simulink model "IEEE_10_CIG_39bus"  (R2023b)
settings: Solver=ode23tb  StartTime=0.0  StopTime=10  MaxStep=1/60  RelTol=1e-2  AbsTol=1e-1  EnableMultiTasking=on
PreLoadFcn:
  | NE39bus_data;
  | PSSMODEL=1;
  | LPSS=0;
  | WAPSS=0;
  | WAPSS2=0;
undefined symbols (not defined in the file): D1, deg, Delta, kp, line, P_base, Pmax, Pmin, s, Udc, V_m
libraries: spsThreePhaseVIMeasurementLib x40, spsThreePhasePISectionLineLib x34, spsThreePhaseParallelRLCLoadLib x19, spsThreePhaseTransformerTwoWindingsLib x13, spsLoadFlowBusLib x10, spsMeanLib x10, spsPowerPositiveSequenceLib x10, spsDCVoltageSourceLib x10, spsUniversalBridgeLib x10, spsThreePhaseSeriesRLCBranchLib x2, spspowerguiLib x1
(part 2 of 2)

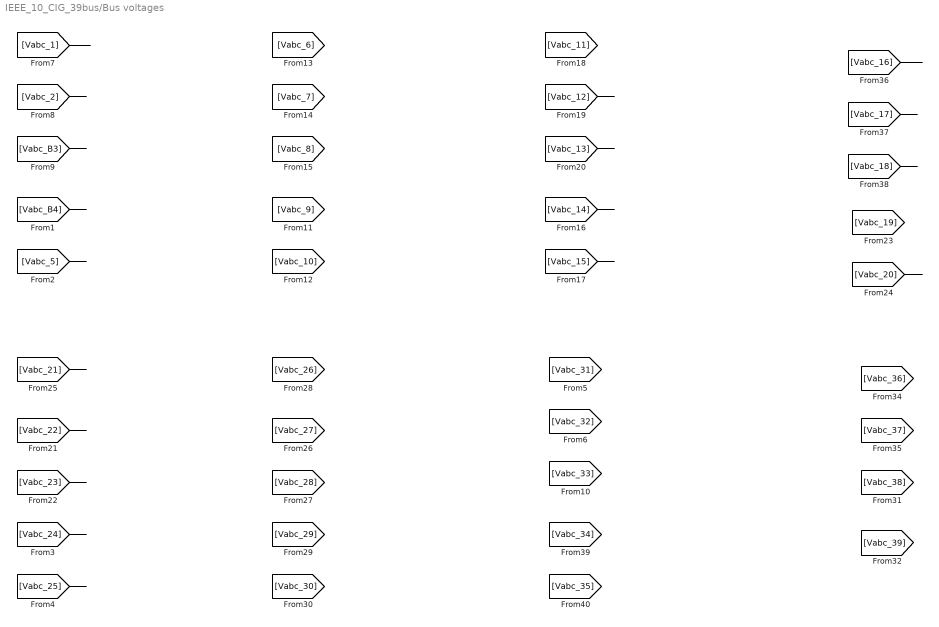
== system IEEE_10_CIG_39bus/Bus voltages ==
  wires:
  [Vabc_1] -> ?
  [Vabc_2] -> ?
  [Vabc_B3] -> ?
  [Vabc_B4] -> ?
  [Vabc_5] -> ?
  [Vabc_24] -> ?
  [Vabc_25] -> ?
  [Vabc_12] -> ?
  [Vabc_13] -> ?
  [Vabc_14] -> ?
  [Vabc_15] -> ?
  [Vabc_20] -> ?
  [Vabc_21] -> ?
  [Vabc_22] -> ?
  [Vabc_23] -> ?
  [Vabc_16] -> ?
  [Vabc_17] -> ?
  [Vabc_18] -> ?

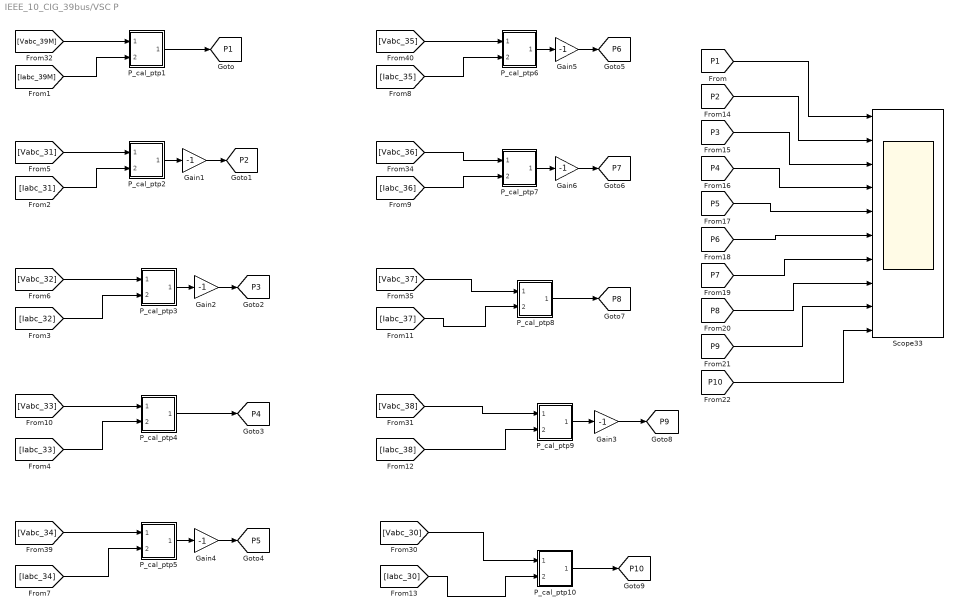
== system IEEE_10_CIG_39bus/VSC P ==
  Gain{1..6} (6 alike) : Gain  Gain=-1
  P_cal_ptp1 : Subsystem
  P_cal_ptp10 : Subsystem
  P_cal_ptp2 : Subsystem
  P_cal_ptp3 : Subsystem
  P_cal_ptp4 : Subsystem
  P_cal_ptp5 : Subsystem
  P_cal_ptp6 : Subsystem
  P_cal_ptp7 : Subsystem
  P_cal_ptp8 : Subsystem
  P_cal_ptp9 : Subsystem
  Scope33 : Scope  NumInputPorts=10
  tag scope: P10=global, P1=global, P2=global, P3=global, P4=global, P5=global, P6=global, P7=global, P8=global, P9=global
  wires:
  [Vabc_39M] -> P_cal_ptp1/1(In2)
  [Iabc_39M] -> P_cal_ptp1/2(In1)
  [Vabc_31] -> P_cal_ptp2/1(In2)
  [Iabc_31] -> P_cal_ptp2/2(In1)
  P_cal_ptp1/1(Out1) -> [P1]
  P_cal_ptp2/1(Out1) -> Gain1/1
  Gain1/1 -> [P2]
  [Vabc_32] -> P_cal_ptp3/1(In2)
  P_cal_ptp3/1(Out1) -> Gain2/1
  [Iabc_32] -> P_cal_ptp3/2(In1)
  Gain2/1 -> [P3]
  [Vabc_33] -> P_cal_ptp4/1(In2)
  [Iabc_33] -> P_cal_ptp4/2(In1)
  P_cal_ptp4/1(Out1) -> [P4]
  [Vabc_34] -> P_cal_ptp5/1(In2)
  P_cal_ptp5/1(Out1) -> Gain4/1
  [Iabc_34] -> P_cal_ptp5/2(In1)
  Gain4/1 -> [P5]
  [Vabc_35] -> P_cal_ptp6/1(In2)
  P_cal_ptp6/1(Out1) -> Gain5/1
  [Iabc_35] -> P_cal_ptp6/2(In1)
  Gain5/1 -> [P6]
  [Vabc_36] -> P_cal_ptp7/1(In2)
  P_cal_ptp7/1(Out1) -> Gain6/1
  [Iabc_36] -> P_cal_ptp7/2(In1)
  Gain6/1 -> [P7]
  [Iabc_37] -> P_cal_ptp8/2(In1)
  [Vabc_37] -> P_cal_ptp8/1(In2)
  P_cal_ptp8/1(Out1) -> [P8]
  [Vabc_38] -> P_cal_ptp9/1(In2)
  [Iabc_38] -> P_cal_ptp9/2(In1)
  P_cal_ptp10/1(Out1) -> [P10]
  [Vabc_30] -> P_cal_ptp10/1(In2)
  [Iabc_30] -> P_cal_ptp10/2(In1)
  [P1] -> Scope33/1
  [P2] -> Scope33/2
  [P3] -> Scope33/3
  [P4] -> Scope33/4
  [P5] -> Scope33/5
  [P6] -> Scope33/6
  [P7] -> Scope33/7
  [P8] -> Scope33/8
  [P9] -> Scope33/9
  [P10] -> Scope33/10
  P_cal_ptp9/1(Out1) -> Gain3/1
  Gain3/1 -> [P9]

== system IEEE_10_CIG_39bus/VSC1 ==
  DC Voltage Source2 : spsDCVoltageSourceLib/DC Voltage Source  Amplitude=Udc(1)  Measurements=None
  Memory2 : Memory
  Subsystem3 : Subsystem
  VSC1 : spsUniversalBridgeLib/Universal Bridge  Arms=3  SnubberResistance=1e5  SnubberCapacitance=inf  Device=Average-model based VSC  Ron=1e-3  Lon=0  ForwardVoltages="[  0  0  ]"  ForwardVoltage=0  GTOparameters=[ 10e-6 , 20e-6 ]  IGBTparameters=[ 1e-6 , 2e-6 ]  Measurements=None  Measurements_2=None  converterType=Rectifier
  Vref1 : Constant  Value=0
  A : PMIOPort  Side=Left
  B : PMIOPort  Port=2  Side=Left
  C : PMIOPort  Port=3  Side=Left
  wires:
  Subsystem3/2(Out2) -> [delta_P1]
  Memory2/1 -> VSC1/1
  [P1] -> Subsystem3/1(P2)
  Vref1/1 -> Subsystem3/2(delta)
  Subsystem3/1(Out1) -> Memory2/1
  connections:
  VSC1/LConn2 -- B/RConn1
  VSC1/RConn1 -- DC Voltage Source2/RConn1
  VSC1/RConn2 -- DC Voltage Source2/LConn1
  VSC1/LConn1 -- A/RConn1
  VSC1/LConn3 -- C/RConn1

== system IEEE_10_CIG_39bus/VSC2 ==
  DC Voltage Source1 : spsDCVoltageSourceLib/DC Voltage Source  Amplitude=Udc(2)  Measurements=None
  Memory1 : Memory
  Subsystem1 : Subsystem
  VSC2 : spsUniversalBridgeLib/Universal Bridge  Arms=3  SnubberResistance=1e5  SnubberCapacitance=inf  Device=Average-model based VSC  Ron=1e-3  Lon=0  ForwardVoltages="[  0  0  ]"  ForwardVoltage=0  GTOparameters=[ 10e-6 , 20e-6 ]  IGBTparameters=[ 1e-6 , 2e-6 ]  Measurements=None  Measurements_2=None  converterType=Rectifier
  Vref2 : Constant  Value=0
  A : PMIOPort  Side=Left
  B : PMIOPort  Port=2  Side=Left
  C : PMIOPort  Port=3  Side=Left
  wires:
  Subsystem1/2(Out2) -> [delta_P2]
  Subsystem1/1(Out1) -> Memory1/1
  Vref2/1 -> Subsystem1/2(delta)
  [P2] -> Subsystem1/1(P2)
  Memory1/1 -> VSC2/1
  connections:
  VSC2/LConn2 -- B/RConn1
  VSC2/RConn2 -- DC Voltage Source1/LConn1
  VSC2/RConn1 -- DC Voltage Source1/RConn1
  VSC2/LConn3 -- C/RConn1
  VSC2/LConn1 -- A/RConn1

== system IEEE_10_CIG_39bus/VSC3 ==
  DC Voltage Source3 : spsDCVoltageSourceLib/DC Voltage Source  Amplitude=Udc(3)  Measurements=None
  Memory3 : Memory
  Subsystem2 : Subsystem
  VSC3 : spsUniversalBridgeLib/Universal Bridge  Arms=3  SnubberResistance=1e5  SnubberCapacitance=inf  Device=Average-model based VSC  Ron=1e-3  Lon=0  ForwardVoltages="[  0  0  ]"  ForwardVoltage=0  GTOparameters=[ 10e-6 , 20e-6 ]  IGBTparameters=[ 1e-6 , 2e-6 ]  Measurements=None  Measurements_2=None  converterType=Rectifier
  Vref3 : Constant  Value=0
  A : PMIOPort  Side=Left
  B : PMIOPort  Port=2  Side=Left
  C : PMIOPort  Port=3  Side=Left
  wires:
  Subsystem2/1(Out1) -> Memory3/1
  Subsystem2/2(Out2) -> [delta_P3]
  [P3] -> Subsystem2/1(P2)
  Vref3/1 -> Subsystem2/2(delta)
  Memory3/1 -> VSC3/1
  connections:
  VSC3/RConn2 -- DC Voltage Source3/LConn1
  VSC3/RConn1 -- DC Voltage Source3/RConn1
  VSC3/LConn1 -- A/RConn1
  VSC3/LConn2 -- B/RConn1
  VSC3/LConn3 -- C/RConn1

== system IEEE_10_CIG_39bus/vsc10 ==
  DC Voltage Source4 : spsDCVoltageSourceLib/DC Voltage Source  Amplitude=Udc(10)  Measurements=None
  Memory4 : Memory
  Subsystem4 : Subsystem
  VSC8 : spsUniversalBridgeLib/Universal Bridge  Arms=3  SnubberResistance=1e5  SnubberCapacitance=inf  Device=Average-model based VSC  Ron=1e-3  Lon=0  ForwardVoltages="[  0  0  ]"  ForwardVoltage=0  GTOparameters=[ 10e-6 , 20e-6 ]  IGBTparameters=[ 1e-6 , 2e-6 ]  Measurements=None  Measurements_2=None  converterType=Rectifier
  Vref4 : Constant  Value=0
  A : PMIOPort  Side=Left
  B : PMIOPort  Port=2  Side=Left
  C : PMIOPort  Port=3  Side=Left
  wires:
  Subsystem4/1(Out1) -> Memory4/1
  Vref4/1 -> Subsystem4/2(delta)
  [P10] -> Subsystem4/1(P2)
  Memory4/1 -> VSC8/1
  Subsystem4/2(Out2) -> [delta_P10]
  connections:
  VSC8/LConn1 -- A/RConn1
  VSC8/RConn2 -- DC Voltage Source4/LConn1
  VSC8/RConn1 -- DC Voltage Source4/RConn1
  VSC8/LConn2 -- B/RConn1
  VSC8/LConn3 -- C/RConn1

== system IEEE_10_CIG_39bus/vsc4 ==
  DC Voltage Source4 : spsDCVoltageSourceLib/DC Voltage Source  Amplitude=Udc(4)  Measurements=None
  Memory4 : Memory
  Subsystem4 : Subsystem
  VSC4 : spsUniversalBridgeLib/Universal Bridge  Arms=3  SnubberResistance=1e5  SnubberCapacitance=inf  Device=Average-model based VSC  Ron=1e-3  Lon=0  ForwardVoltages="[  0  0  ]"  ForwardVoltage=0  GTOparameters=[ 10e-6 , 20e-6 ]  IGBTparameters=[ 1e-6 , 2e-6 ]  Measurements=None  Measurements_2=None  converterType=Rectifier
  Vref4 : Constant  Value=0
  A : PMIOPort  Side=Left
  B : PMIOPort  Port=2  Side=Left
  C : PMIOPort  Port=3  Side=Left
  wires:
  Subsystem4/1(Out1) -> Memory4/1
  Vref4/1 -> Subsystem4/2(delta)
  [P4] -> Subsystem4/1(P2)
  Memory4/1 -> VSC4/1
  Subsystem4/2(Out2) -> [delta_P4]
  connections:
  VSC4/LConn1 -- A/RConn1
  VSC4/RConn2 -- DC Voltage Source4/LConn1
  VSC4/RConn1 -- DC Voltage Source4/RConn1
  VSC4/LConn2 -- B/RConn1
  VSC4/LConn3 -- C/RConn1

== system IEEE_10_CIG_39bus/vsc5 ==
  DC Voltage Source4 : spsDCVoltageSourceLib/DC Voltage Source  Amplitude=Udc(5)  Measurements=None
  Memory4 : Memory
  Subsystem4 : Subsystem
  VSC5 : spsUniversalBridgeLib/Universal Bridge  Arms=3  SnubberResistance=1e5  SnubberCapacitance=inf  Device=Average-model based VSC  Ron=1e-3  Lon=0  ForwardVoltages="[  0  0  ]"  ForwardVoltage=0  GTOparameters=[ 10e-6 , 20e-6 ]  IGBTparameters=[ 1e-6 , 2e-6 ]  Measurements=None  Measurements_2=None  converterType=Rectifier
  Vref4 : Constant  Value=0
  A : PMIOPort  Side=Left
  B : PMIOPort  Port=2  Side=Left
  C : PMIOPort  Port=3  Side=Left
  wires:
  Subsystem4/1(Out1) -> Memory4/1
  Vref4/1 -> Subsystem4/2(delta)
  [P5] -> Subsystem4/1(P2)
  Memory4/1 -> VSC5/1
  Subsystem4/2(Out2) -> [delta_P5]
  connections:
  VSC5/LConn1 -- A/RConn1
  VSC5/RConn2 -- DC Voltage Source4/LConn1
  VSC5/RConn1 -- DC Voltage Source4/RConn1
  VSC5/LConn2 -- B/RConn1
  VSC5/LConn3 -- C/RConn1

== system IEEE_10_CIG_39bus/vsc6 ==
  DC Voltage Source4 : spsDCVoltageSourceLib/DC Voltage Source  Amplitude=Udc(6)  Measurements=None
  Memory4 : Memory
  Subsystem4 : Subsystem
  VSC6 : spsUniversalBridgeLib/Universal Bridge  Arms=3  SnubberResistance=1e5  SnubberCapacitance=inf  Device=Average-model based VSC  Ron=1e-3  Lon=0  ForwardVoltages="[  0  0  ]"  ForwardVoltage=0  GTOparameters=[ 10e-6 , 20e-6 ]  IGBTparameters=[ 1e-6 , 2e-6 ]  Measurements=None  Measurements_2=None  converterType=Rectifier
  Vref4 : Constant  Value=0
  A : PMIOPort  Side=Left
  B : PMIOPort  Port=2  Side=Left
  C : PMIOPort  Port=3  Side=Left
  wires:
  Subsystem4/1(Out1) -> Memory4/1
  Vref4/1 -> Subsystem4/2(delta)
  [P6] -> Subsystem4/1(P2)
  Memory4/1 -> VSC6/1
  Subsystem4/2(Out2) -> [delta_P6]
  connections:
  VSC6/LConn1 -- A/RConn1
  VSC6/RConn2 -- DC Voltage Source4/LConn1
  VSC6/RConn1 -- DC Voltage Source4/RConn1
  VSC6/LConn2 -- B/RConn1
  VSC6/LConn3 -- C/RConn1

== system IEEE_10_CIG_39bus/vsc7 ==
  DC Voltage Source4 : spsDCVoltageSourceLib/DC Voltage Source  Amplitude=Udc(7)  Measurements=None
  Memory4 : Memory
  Subsystem4 : Subsystem
  VSC7 : spsUniversalBridgeLib/Universal Bridge  Arms=3  SnubberResistance=1e5  SnubberCapacitance=inf  Device=Average-model based VSC  Ron=1e-3  Lon=0  ForwardVoltages="[  0  0  ]"  ForwardVoltage=0  GTOparameters=[ 10e-6 , 20e-6 ]  IGBTparameters=[ 1e-6 , 2e-6 ]  Measurements=None  Measurements_2=None  converterType=Rectifier
  Vref4 : Constant  Value=0
  A : PMIOPort  Side=Left
  B : PMIOPort  Port=2  Side=Left
  C : PMIOPort  Port=3  Side=Left
  wires:
  Subsystem4/1(Out1) -> Memory4/1
  Vref4/1 -> Subsystem4/2(delta)
  [P7] -> Subsystem4/1(P2)
  Memory4/1 -> VSC7/1
  Subsystem4/2(Out2) -> [delta_P7]
  connections:
  VSC7/LConn1 -- A/RConn1
  VSC7/RConn2 -- DC Voltage Source4/LConn1
  VSC7/RConn1 -- DC Voltage Source4/RConn1
  VSC7/LConn2 -- B/RConn1
  VSC7/LConn3 -- C/RConn1

== system IEEE_10_CIG_39bus/vsc8 ==
  DC Voltage Source4 : spsDCVoltageSourceLib/DC Voltage Source  Amplitude=Udc(8)  Measurements=None
  Memory4 : Memory
  Subsystem4 : Subsystem
  VSC8 : spsUniversalBridgeLib/Universal Bridge  Arms=3  SnubberResistance=1e5  SnubberCapacitance=inf  Device=Average-model based VSC  Ron=1e-3  Lon=0  ForwardVoltages="[  0  0  ]"  ForwardVoltage=0  GTOparameters=[ 10e-6 , 20e-6 ]  IGBTparameters=[ 1e-6 , 2e-6 ]  Measurements=None  Measurements_2=None  converterType=Rectifier
  Vref4 : Constant  Value=0
  A : PMIOPort  Side=Left
  B : PMIOPort  Port=2  Side=Left
  C : PMIOPort  Port=3  Side=Left
  wires:
  Subsystem4/1(Out1) -> Memory4/1
  Vref4/1 -> Subsystem4/2(delta)
  [P8] -> Subsystem4/1(P2)
  Memory4/1 -> VSC8/1
  Subsystem4/2(Out2) -> [delta_P8]
  connections:
  VSC8/LConn1 -- A/RConn1
  VSC8/RConn2 -- DC Voltage Source4/LConn1
  VSC8/RConn1 -- DC Voltage Source4/RConn1
  VSC8/LConn2 -- B/RConn1
  VSC8/LConn3 -- C/RConn1

== system IEEE_10_CIG_39bus/vsc9 ==
  DC Voltage Source4 : spsDCVoltageSourceLib/DC Voltage Source  Amplitude=Udc(9)  Measurements=None
  Memory4 : Memory
  Subsystem4 : Subsystem
  VSC5 : spsUniversalBridgeLib/Universal Bridge  Arms=3  SnubberResistance=1e5  SnubberCapacitance=inf  Device=Average-model based VSC  Ron=1e-3  Lon=0  ForwardVoltages="[  0  0  ]"  ForwardVoltage=0  GTOparameters=[ 10e-6 , 20e-6 ]  IGBTparameters=[ 1e-6 , 2e-6 ]  Measurements=None  Measurements_2=None  converterType=Rectifier
  Vref4 : Constant  Value=0
  A : PMIOPort  Side=Left
  B : PMIOPort  Port=2  Side=Left
  C : PMIOPort  Port=3  Side=Left
  wires:
  Subsystem4/1(Out1) -> Memory4/1
  Vref4/1 -> Subsystem4/2(delta)
  [P9] -> Subsystem4/1(P2)
  Memory4/1 -> VSC5/1
  Subsystem4/2(Out2) -> [delta_P9]
  connections:
  VSC5/LConn1 -- A/RConn1
  VSC5/RConn2 -- DC Voltage Source4/LConn1
  VSC5/RConn1 -- DC Voltage Source4/RConn1
  VSC5/LConn2 -- B/RConn1
  VSC5/LConn3 -- C/RConn1

== system IEEE_10_CIG_39bus/VSC P/P_cal_ptp1 ==
  In2 : Inport
  In1 : Inport  Port=2
  Demux1 : Demux  Outputs=3
  Demux2 : Demux  Outputs=3
  Divide1 : Product  Inputs=**
  Divide2 : Product  Inputs=**
  Divide3 : Product  Inputs=**
  Gain : Gain  Gain=-1/3
  Gain1 : Gain  Gain=-1/3
  Gain2 : Gain  Gain=-1/3
  Mean : spsMeanLib/Mean  Freq=60  Vinit=P_base(1)  Ts=0
  Mux : Mux  Inputs=3
  Power (Positive-Sequence)1 : spsPowerPositiveSequenceLib/Power (Positive-Sequence)  Freq=60  Vinit=[0, 0]  Iinit=[0, 0]  Ts=1e-4
  Subtract1 : Sum  Inputs=+++
  Sum : Sum  Inputs=|+-
  Sum1 : Sum  Inputs=|+-
  Sum2 : Sum  Inputs=|+-
  Out1 : Outport
  wires:
  Sum2/1 -> Gain2/1
  Demux1/3 -> Sum2/1, Sum1/2
  Demux1/1 -> Sum2/2, Sum/1
  Demux1/2 -> Sum1/1, Sum/2
  Demux2/2 -> Divide1/1
  Gain1/1 -> Divide2/2, Mux/3
  Divide1/1 -> Subtract1/2
  Divide3/1 -> Subtract1/1
  Sum1/1 -> Gain1/1
  In1/1 -> Power (Positive-Sequence)1/2, Demux2/1
  Divide2/1 -> Subtract1/3
  Demux2/3 -> Divide2/1
  Demux2/1 -> Divide3/1
  Gain/1 -> Mux/2, Divide1/2
  Sum/1 -> Gain/1
  Gain2/1 -> Mux/1, Divide3/2
  In2/1 -> Demux1/1
  Mean/1 -> Out1/1
  Mux/1 -> Power (Positive-Sequence)1/1
  Power (Positive-Sequence)1/1 -> Mean/1

== system IEEE_10_CIG_39bus/VSC P/P_cal_ptp10 ==
  In2 : Inport
  In1 : Inport  Port=2
  Demux1 : Demux  Outputs=3
  Demux2 : Demux  Outputs=3
  Divide1 : Product  Inputs=**
  Divide2 : Product  Inputs=**
  Divide3 : Product  Inputs=**
  Gain : Gain  Gain=-1/3
  Gain1 : Gain  Gain=-1/3
  Gain2 : Gain  Gain=-1/3
  Mean : spsMeanLib/Mean  Freq=60  Vinit=P_base(10)  Ts=0
  Mux : Mux  Inputs=3
  Power (Positive-Sequence)1 : spsPowerPositiveSequenceLib/Power (Positive-Sequence)  Freq=60  Vinit=[0, 0]  Iinit=[0, 0]  Ts=1e-4
  Subtract1 : Sum  Inputs=+++
  Sum : Sum  Inputs=|+-
  Sum1 : Sum  Inputs=|+-
  Sum2 : Sum  Inputs=|+-
  Out1 : Outport
  wires:
  Sum2/1 -> Gain2/1
  Demux1/3 -> Sum2/1, Sum1/2
  Demux1/1 -> Sum2/2, Sum/1
  Demux1/2 -> Sum1/1, Sum/2
  Demux2/2 -> Divide1/1
  Gain1/1 -> Divide2/2, Mux/3
  Divide1/1 -> Subtract1/2
  Divide3/1 -> Subtract1/1
  Sum1/1 -> Gain1/1
  In1/1 -> Power (Positive-Sequence)1/2, Demux2/1
  Divide2/1 -> Subtract1/3
  Demux2/3 -> Divide2/1
  Demux2/1 -> Divide3/1
  Gain/1 -> Mux/2, Divide1/2
  Sum/1 -> Gain/1
  Gain2/1 -> Mux/1, Divide3/2
  In2/1 -> Demux1/1
  Mean/1 -> Out1/1
  Mux/1 -> Power (Positive-Sequence)1/1
  Power (Positive-Sequence)1/1 -> Mean/1

== system IEEE_10_CIG_39bus/VSC P/P_cal_ptp2 ==
  In2 : Inport
  In1 : Inport  Port=2
  Demux1 : Demux  Outputs=3
  Demux2 : Demux  Outputs=3
  Divide1 : Product  Inputs=**
  Divide2 : Product  Inputs=**
  Divide3 : Product  Inputs=**
  Gain : Gain  Gain=-1/3
  Gain1 : Gain  Gain=-1/3
  Gain2 : Gain  Gain=-1/3
  Mean : spsMeanLib/Mean  Freq=60  Vinit=-P_base(2)  Ts=0
  Mux : Mux  Inputs=3
  Power (Positive-Sequence)1 : spsPowerPositiveSequenceLib/Power (Positive-Sequence)  Freq=60  Vinit=[0, 0]  Iinit=[0, 0]  Ts=1e-4
  Subtract1 : Sum  Inputs=+++
  Sum : Sum  Inputs=|+-
  Sum1 : Sum  Inputs=|+-
  Sum2 : Sum  Inputs=|+-
  Out1 : Outport
  wires:
  Sum2/1 -> Gain2/1
  Demux1/3 -> Sum2/1, Sum1/2
  Demux1/1 -> Sum2/2, Sum/1
  Demux1/2 -> Sum1/1, Sum/2
  Demux2/2 -> Divide1/1
  Gain1/1 -> Divide2/2, Mux/3
  Divide1/1 -> Subtract1/2
  Divide3/1 -> Subtract1/1
  Sum1/1 -> Gain1/1
  In1/1 -> Power (Positive-Sequence)1/2, Demux2/1
  Divide2/1 -> Subtract1/3
  Demux2/3 -> Divide2/1
  Demux2/1 -> Divide3/1
  Gain/1 -> Mux/2, Divide1/2
  Sum/1 -> Gain/1
  Gain2/1 -> Mux/1, Divide3/2
  In2/1 -> Demux1/1
  Mean/1 -> Out1/1
  Mux/1 -> Power (Positive-Sequence)1/1
  Power (Positive-Sequence)1/1 -> Mean/1

== system IEEE_10_CIG_39bus/VSC P/P_cal_ptp3 ==
  In2 : Inport
  In1 : Inport  Port=2
  Demux1 : Demux  Outputs=3
  Demux2 : Demux  Outputs=3
  Divide1 : Product  Inputs=**
  Divide2 : Product  Inputs=**
  Divide3 : Product  Inputs=**
  Gain : Gain  Gain=-1/3
  Gain1 : Gain  Gain=-1/3
  Gain2 : Gain  Gain=-1/3
  Mean : spsMeanLib/Mean  Freq=60  Vinit=-P_base(3)  Ts=0
  Mux : Mux  Inputs=3
  Power (Positive-Sequence)1 : spsPowerPositiveSequenceLib/Power (Positive-Sequence)  Freq=60  Vinit=[0, 0]  Iinit=[0, 0]  Ts=1e-4
  Subtract1 : Sum  Inputs=+++
  Sum : Sum  Inputs=|+-
  Sum1 : Sum  Inputs=|+-
  Sum2 : Sum  Inputs=|+-
  Out1 : Outport
  wires:
  Sum2/1 -> Gain2/1
  Demux1/3 -> Sum2/1, Sum1/2
  Demux1/1 -> Sum2/2, Sum/1
  Demux1/2 -> Sum1/1, Sum/2
  Demux2/2 -> Divide1/1
  Gain1/1 -> Divide2/2, Mux/3
  Divide1/1 -> Subtract1/2
  Divide3/1 -> Subtract1/1
  Sum1/1 -> Gain1/1
  In1/1 -> Power (Positive-Sequence)1/2, Demux2/1
  Divide2/1 -> Subtract1/3
  Demux2/3 -> Divide2/1
  Demux2/1 -> Divide3/1
  Gain/1 -> Mux/2, Divide1/2
  Sum/1 -> Gain/1
  Gain2/1 -> Mux/1, Divide3/2
  In2/1 -> Demux1/1
  Mean/1 -> Out1/1
  Mux/1 -> Power (Positive-Sequence)1/1
  Power (Positive-Sequence)1/1 -> Mean/1

== system IEEE_10_CIG_39bus/VSC P/P_cal_ptp4 ==
  In2 : Inport
  In1 : Inport  Port=2
  Demux1 : Demux  Outputs=3
  Demux2 : Demux  Outputs=3
  Divide1 : Product  Inputs=**
  Divide2 : Product  Inputs=**
  Divide3 : Product  Inputs=**
  Gain : Gain  Gain=-1/3
  Gain1 : Gain  Gain=-1/3
  Gain2 : Gain  Gain=-1/3
  Mean : spsMeanLib/Mean  Freq=60  Vinit=P_base(4)  Ts=0
  Mux : Mux  Inputs=3
  Power (Positive-Sequence)1 : spsPowerPositiveSequenceLib/Power (Positive-Sequence)  Freq=60  Vinit=[0, 0]  Iinit=[0, 0]  Ts=1e-4
  Subtract1 : Sum  Inputs=+++
  Sum : Sum  Inputs=|+-
  Sum1 : Sum  Inputs=|+-
  Sum2 : Sum  Inputs=|+-
  Out1 : Outport
  wires:
  Sum2/1 -> Gain2/1
  Demux1/3 -> Sum2/1, Sum1/2
  Demux1/1 -> Sum2/2, Sum/1
  Demux1/2 -> Sum1/1, Sum/2
  Demux2/2 -> Divide1/1
  Gain1/1 -> Divide2/2, Mux/3
  Divide1/1 -> Subtract1/2
  Divide3/1 -> Subtract1/1
  Sum1/1 -> Gain1/1
  In1/1 -> Power (Positive-Sequence)1/2, Demux2/1
  Divide2/1 -> Subtract1/3
  Demux2/3 -> Divide2/1
  Demux2/1 -> Divide3/1
  Gain/1 -> Mux/2, Divide1/2
  Sum/1 -> Gain/1
  Gain2/1 -> Mux/1, Divide3/2
  In2/1 -> Demux1/1
  Mean/1 -> Out1/1
  Mux/1 -> Power (Positive-Sequence)1/1
  Power (Positive-Sequence)1/1 -> Mean/1

== system IEEE_10_CIG_39bus/VSC P/P_cal_ptp5 ==
  In2 : Inport
  In1 : Inport  Port=2
  Demux1 : Demux  Outputs=3
  Demux2 : Demux  Outputs=3
  Divide1 : Product  Inputs=**
  Divide2 : Product  Inputs=**
  Divide3 : Product  Inputs=**
  Gain : Gain  Gain=-1/3
  Gain1 : Gain  Gain=-1/3
  Gain2 : Gain  Gain=-1/3
  Mean : spsMeanLib/Mean  Freq=60  Vinit=-P_base(5)  Ts=0
  Mux : Mux  Inputs=3
  Power (Positive-Sequence)1 : spsPowerPositiveSequenceLib/Power (Positive-Sequence)  Freq=60  Vinit=[0, 0]  Iinit=[0, 0]  Ts=1e-4
  Subtract1 : Sum  Inputs=+++
  Sum : Sum  Inputs=|+-
  Sum1 : Sum  Inputs=|+-
  Sum2 : Sum  Inputs=|+-
  Out1 : Outport
  wires:
  Sum2/1 -> Gain2/1
  Demux1/3 -> Sum2/1, Sum1/2
  Demux1/1 -> Sum2/2, Sum/1
  Demux1/2 -> Sum1/1, Sum/2
  Demux2/2 -> Divide1/1
  Gain1/1 -> Divide2/2, Mux/3
  Divide1/1 -> Subtract1/2
  Divide3/1 -> Subtract1/1
  Sum1/1 -> Gain1/1
  In1/1 -> Power (Positive-Sequence)1/2, Demux2/1
  Divide2/1 -> Subtract1/3
  Demux2/3 -> Divide2/1
  Demux2/1 -> Divide3/1
  Gain/1 -> Mux/2, Divide1/2
  Sum/1 -> Gain/1
  Gain2/1 -> Mux/1, Divide3/2
  In2/1 -> Demux1/1
  Mean/1 -> Out1/1
  Mux/1 -> Power (Positive-Sequence)1/1
  Power (Positive-Sequence)1/1 -> Mean/1

== system IEEE_10_CIG_39bus/VSC P/P_cal_ptp6 ==
  In2 : Inport
  In1 : Inport  Port=2
  Demux1 : Demux  Outputs=3
  Demux2 : Demux  Outputs=3
  Divide1 : Product  Inputs=**
  Divide2 : Product  Inputs=**
  Divide3 : Product  Inputs=**
  Gain : Gain  Gain=-1/3
  Gain1 : Gain  Gain=-1/3
  Gain2 : Gain  Gain=-1/3
  Mean : spsMeanLib/Mean  Freq=60  Vinit=-P_base(6)  Ts=0
  Mux : Mux  Inputs=3
  Power (Positive-Sequence)1 : spsPowerPositiveSequenceLib/Power (Positive-Sequence)  Freq=60  Vinit=[0, 0]  Iinit=[0, 0]  Ts=1e-4
  Subtract1 : Sum  Inputs=+++
  Sum : Sum  Inputs=|+-
  Sum1 : Sum  Inputs=|+-
  Sum2 : Sum  Inputs=|+-
  Out1 : Outport
  wires:
  Sum2/1 -> Gain2/1
  Demux1/3 -> Sum2/1, Sum1/2
  Demux1/1 -> Sum2/2, Sum/1
  Demux1/2 -> Sum1/1, Sum/2
  Demux2/2 -> Divide1/1
  Gain1/1 -> Divide2/2, Mux/3
  Divide1/1 -> Subtract1/2
  Divide3/1 -> Subtract1/1
  Sum1/1 -> Gain1/1
  In1/1 -> Power (Positive-Sequence)1/2, Demux2/1
  Divide2/1 -> Subtract1/3
  Demux2/3 -> Divide2/1
  Demux2/1 -> Divide3/1
  Gain/1 -> Mux/2, Divide1/2
  Sum/1 -> Gain/1
  Gain2/1 -> Mux/1, Divide3/2
  In2/1 -> Demux1/1
  Mean/1 -> Out1/1
  Mux/1 -> Power (Positive-Sequence)1/1
  Power (Positive-Sequence)1/1 -> Mean/1

== system IEEE_10_CIG_39bus/VSC P/P_cal_ptp7 ==
  In2 : Inport
  In1 : Inport  Port=2
  Demux1 : Demux  Outputs=3
  Demux2 : Demux  Outputs=3
  Divide1 : Product  Inputs=**
  Divide2 : Product  Inputs=**
  Divide3 : Product  Inputs=**
  Gain : Gain  Gain=-1/3
  Gain1 : Gain  Gain=-1/3
  Gain2 : Gain  Gain=-1/3
  Mean : spsMeanLib/Mean  Freq=60  Vinit=-P_base(7)  Ts=0
  Mux : Mux  Inputs=3
  Power (Positive-Sequence)1 : spsPowerPositiveSequenceLib/Power (Positive-Sequence)  Freq=60  Vinit=[0, 0]  Iinit=[0, 0]  Ts=1e-4
  Subtract1 : Sum  Inputs=+++
  Sum : Sum  Inputs=|+-
  Sum1 : Sum  Inputs=|+-
  Sum2 : Sum  Inputs=|+-
  Out1 : Outport
  wires:
  Sum2/1 -> Gain2/1
  Demux1/3 -> Sum2/1, Sum1/2
  Demux1/1 -> Sum2/2, Sum/1
  Demux1/2 -> Sum1/1, Sum/2
  Demux2/2 -> Divide1/1
  Gain1/1 -> Divide2/2, Mux/3
  Divide1/1 -> Subtract1/2
  Divide3/1 -> Subtract1/1
  Sum1/1 -> Gain1/1
  In1/1 -> Power (Positive-Sequence)1/2, Demux2/1
  Divide2/1 -> Subtract1/3
  Demux2/3 -> Divide2/1
  Demux2/1 -> Divide3/1
  Gain/1 -> Mux/2, Divide1/2
  Sum/1 -> Gain/1
  Gain2/1 -> Mux/1, Divide3/2
  In2/1 -> Demux1/1
  Mean/1 -> Out1/1
  Mux/1 -> Power (Positive-Sequence)1/1
  Power (Positive-Sequence)1/1 -> Mean/1

== system IEEE_10_CIG_39bus/VSC P/P_cal_ptp8 ==
  In2 : Inport
  In1 : Inport  Port=2
  Demux1 : Demux  Outputs=3
  Demux2 : Demux  Outputs=3
  Divide1 : Product  Inputs=**
  Divide2 : Product  Inputs=**
  Divide3 : Product  Inputs=**
  Gain : Gain  Gain=-1/3
  Gain1 : Gain  Gain=-1/3
  Gain2 : Gain  Gain=-1/3
  Mean : spsMeanLib/Mean  Freq=60  Vinit=P_base(8)  Ts=0
  Mux : Mux  Inputs=3
  Power (Positive-Sequence)1 : spsPowerPositiveSequenceLib/Power (Positive-Sequence)  Freq=60  Vinit=[0, 0]  Iinit=[0, 0]  Ts=1e-4
  Subtract1 : Sum  Inputs=+++
  Sum : Sum  Inputs=|+-
  Sum1 : Sum  Inputs=|+-
  Sum2 : Sum  Inputs=|+-
  Out1 : Outport
  wires:
  Sum2/1 -> Gain2/1
  Demux1/3 -> Sum2/1, Sum1/2
  Demux1/1 -> Sum2/2, Sum/1
  Demux1/2 -> Sum1/1, Sum/2
  Demux2/2 -> Divide1/1
  Gain1/1 -> Divide2/2, Mux/3
  Divide1/1 -> Subtract1/2
  Divide3/1 -> Subtract1/1
  Sum1/1 -> Gain1/1
  In1/1 -> Power (Positive-Sequence)1/2, Demux2/1
  Divide2/1 -> Subtract1/3
  Demux2/3 -> Divide2/1
  Demux2/1 -> Divide3/1
  Gain/1 -> Mux/2, Divide1/2
  Sum/1 -> Gain/1
  Gain2/1 -> Mux/1, Divide3/2
  In2/1 -> Demux1/1
  Mean/1 -> Out1/1
  Mux/1 -> Power (Positive-Sequence)1/1
  Power (Positive-Sequence)1/1 -> Mean/1

== system IEEE_10_CIG_39bus/VSC P/P_cal_ptp9 ==
  In2 : Inport
  In1 : Inport  Port=2
  Demux1 : Demux  Outputs=3
  Demux2 : Demux  Outputs=3
  Divide1 : Product  Inputs=**
  Divide2 : Product  Inputs=**
  Divide3 : Product  Inputs=**
  Gain : Gain  Gain=-1/3
  Gain1 : Gain  Gain=-1/3
  Gain2 : Gain  Gain=-1/3
  Mean : spsMeanLib/Mean  Freq=60  Vinit=-P_base(9)  Ts=0
  Mux : Mux  Inputs=3
  Power (Positive-Sequence)1 : spsPowerPositiveSequenceLib/Power (Positive-Sequence)  Freq=60  Vinit=[0, 0]  Iinit=[0, 0]  Ts=1e-4
  Subtract1 : Sum  Inputs=+++
  Sum : Sum  Inputs=|+-
  Sum1 : Sum  Inputs=|+-
  Sum2 : Sum  Inputs=|+-
  Out1 : Outport
  wires:
  Sum2/1 -> Gain2/1
  Demux1/3 -> Sum2/1, Sum1/2
  Demux1/1 -> Sum2/2, Sum/1
  Demux1/2 -> Sum1/1, Sum/2
  Demux2/2 -> Divide1/1
  Gain1/1 -> Divide2/2, Mux/3
  Divide1/1 -> Subtract1/2
  Divide3/1 -> Subtract1/1
  Sum1/1 -> Gain1/1
  In1/1 -> Power (Positive-Sequence)1/2, Demux2/1
  Divide2/1 -> Subtract1/3
  Demux2/3 -> Divide2/1
  Demux2/1 -> Divide3/1
  Gain/1 -> Mux/2, Divide1/2
  Sum/1 -> Gain/1
  Gain2/1 -> Mux/1, Divide3/2
  In2/1 -> Demux1/1
  Mean/1 -> Out1/1
  Mux/1 -> Power (Positive-Sequence)1/1
  Power (Positive-Sequence)1/1 -> Mean/1

== system IEEE_10_CIG_39bus/VSC1/Subsystem3 ==
  P2 : Inport
  delta : Inport  Port=2
  Add1 : Sum  Inputs=++++
  Clock1 : Clock
  Constant1 : Constant  Value="[0  -2/3*pi   2/3*pi]+deg(1)"
  Constant2 : Constant  Value=0
  Constant3 : Constant  Value=0
  Constant4 : Constant  Value=Pmax(1)
  Constant5 : Constant  Value=Pmin(1)
  Gain : Gain  Gain=kp(1)
  Gain1 : Gain  Gain=[1 1 1]
  Gain2 : Gain  Gain=120*pi*[1 1 1]
  Gain3 : Gain  Gain=V_m(1)
  Gain4 : Gain  Gain=1/P_base(1)
  Gain5 : Gain  Gain=[1 1 1]
  Gain6 : Gain  Gain=-1
  Integrator : Integrator
  Product : Product
  Product1 : Product
  Scope1 : Scope
  Scope2 : Scope
  Scope3 : Scope
  Step : Step  Time=5  SampleTime=0
  Step1 : Step  Time=5  SampleTime=0
  Sum : Sum  Inputs=|+-
  Sum1 : Sum  Inputs=|+-
  Sum2 : Sum  Inputs=|++
  Switch : Switch  Criteria=u2 > Threshold  Threshold=Pmax(1)  SaturateOnIntegerOverflow=off  InputSameDT=off
  Switch1 : Switch  Criteria=u2 > Threshold  Threshold=-Pmin(1)  SaturateOnIntegerOverflow=off  InputSameDT=off
  Trigonometric Function1 : Trigonometry
  Out1 : Outport
  Out2 : Outport  Port=2
  wires:
  Clock1/1 -> Gain2/1
  Constant1/1 -> Add1/2
  Gain2/1 -> Add1/1
  Add1/1 -> Trigonometric Function1/1
  Gain1/1 -> Product/1
  Step/1 -> Product/2
  Product/1 -> Add1/3
  Trigonometric Function1/1 -> Gain3/1
  Gain3/1 -> Out1/1
  Gain/1 -> Scope2/1, Gain1/1
  Integrator/1 -> Gain/1
  P2/1 -> Gain4/1
  delta/1 -> Gain5/1
  Gain5/1 -> Add1/4
  Step1/1 -> Product1/2
  Product1/1 -> Integrator/1
  Constant4/1 -> Sum/1
  Sum/1 -> Switch/1
  Constant2/1 -> Switch/3
  Constant5/1 -> Sum1/1
  Sum1/1 -> Switch1/1
  Gain4/1 -> Gain6/1, Sum1/2, Sum/2, Switch/2
  Constant3/1 -> Switch1/3
  Gain6/1 -> Switch1/2
  Switch/1 -> Scope1/1, Sum2/1
  Switch1/1 -> Scope3/1, Sum2/2
  Sum2/1 -> Out2/1, Product1/1

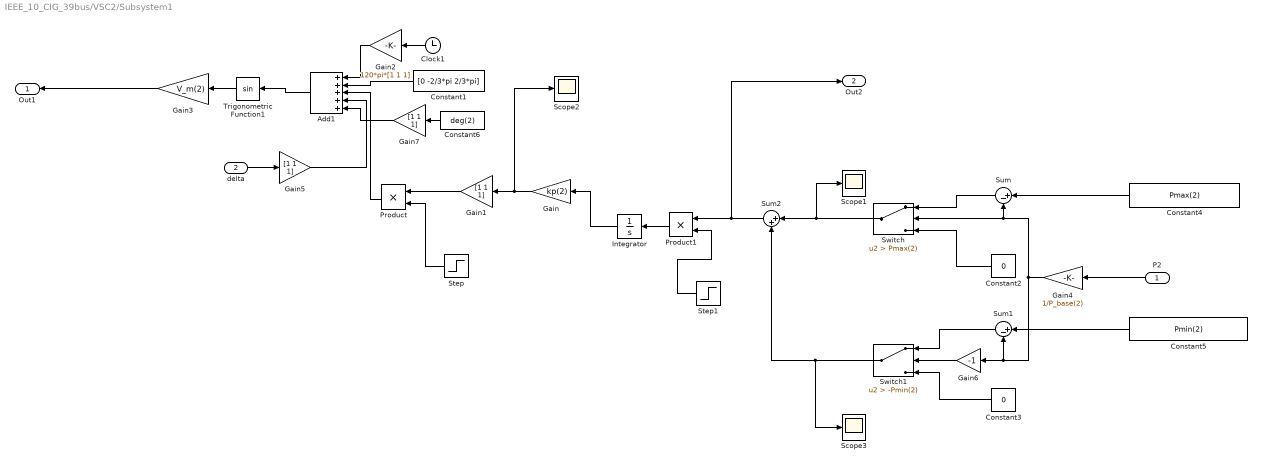
== system IEEE_10_CIG_39bus/VSC2/Subsystem1 ==
  P2 : Inport
  delta : Inport  Port=2
  Add1 : Sum  Inputs=+++++
  Clock1 : Clock
  Constant1 : Constant  Value="[0  -2/3*pi   2/3*pi]"
  Constant2 : Constant  Value=0
  Constant3 : Constant  Value=0
  Constant4 : Constant  Value=Pmax(2)
  Constant5 : Constant  Value=Pmin(2)
  Constant6 : Constant  Value=deg(2)
  Gain : Gain  Gain=kp(2)
  Gain1 : Gain  Gain=[1 1 1]
  Gain2 : Gain  Gain=120*pi*[1 1 1]
  Gain3 : Gain  Gain=V_m(2)
  Gain4 : Gain  Gain=1/P_base(2)
  Gain5 : Gain  Gain=[1 1 1]
  Gain6 : Gain  Gain=-1
  Gain7 : Gain  Gain=[1 1 1]
  Integrator : Integrator
  Product : Product
  Product1 : Product
  Scope1 : Scope
  Scope2 : Scope
  Scope3 : Scope
  Step : Step  Time=5  SampleTime=0
  Step1 : Step  Time=5  SampleTime=0
  Sum : Sum  Inputs=|+-
  Sum1 : Sum  Inputs=|+-
  Sum2 : Sum  Inputs=|++
  Switch : Switch  Criteria=u2 > Threshold  Threshold=Pmax(2)  SaturateOnIntegerOverflow=off  InputSameDT=off
  Switch1 : Switch  Criteria=u2 > Threshold  Threshold=-Pmin(2)  SaturateOnIntegerOverflow=off  InputSameDT=off
  Trigonometric Function1 : Trigonometry
  Out1 : Outport
  Out2 : Outport  Port=2
  wires:
  Clock1/1 -> Gain2/1
  Constant1/1 -> Add1/2
  Gain2/1 -> Add1/1
  Add1/1 -> Trigonometric Function1/1
  Gain1/1 -> Product/1
  Step/1 -> Product/2
  Product/1 -> Add1/3
  Trigonometric Function1/1 -> Gain3/1
  Gain3/1 -> Out1/1
  Gain/1 -> Scope2/1, Gain1/1
  Integrator/1 -> Gain/1
  P2/1 -> Gain4/1
  delta/1 -> Gain5/1
  Gain5/1 -> Add1/4
  Step1/1 -> Product1/2
  Product1/1 -> Integrator/1
  Constant4/1 -> Sum/1
  Sum/1 -> Switch/1
  Constant2/1 -> Switch/3
  Constant5/1 -> Sum1/1
  Sum1/1 -> Switch1/1
  Gain4/1 -> Gain6/1, Sum1/2, Sum/2, Switch/2
  Constant3/1 -> Switch1/3
  Gain6/1 -> Switch1/2
  Switch/1 -> Scope1/1, Sum2/1
  Switch1/1 -> Scope3/1, Sum2/2
  Sum2/1 -> Out2/1, Product1/1
  Constant6/1 -> Gain7/1
  Gain7/1 -> Add1/5

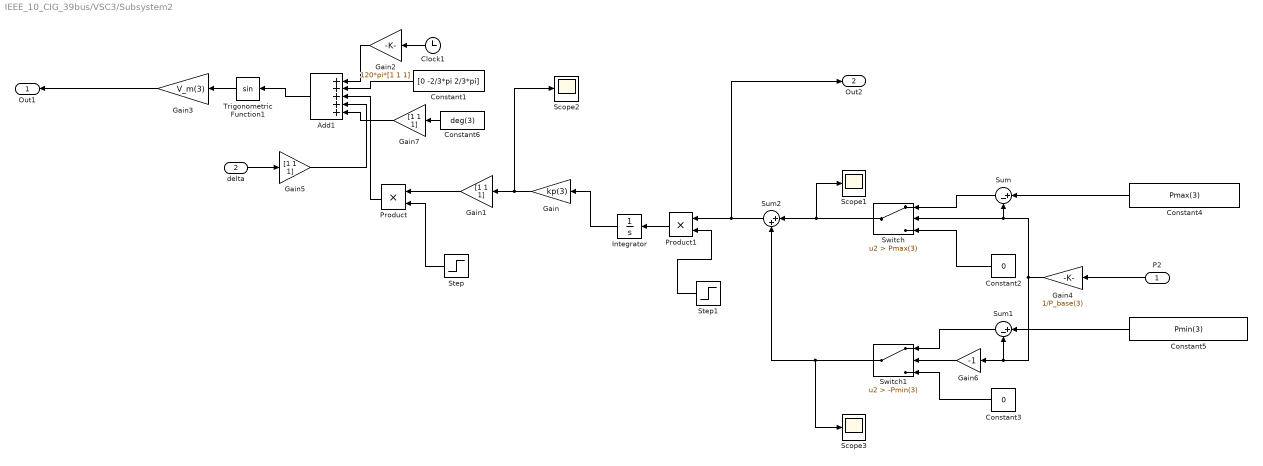
== system IEEE_10_CIG_39bus/VSC3/Subsystem2 ==
  P2 : Inport
  delta : Inport  Port=2
  Add1 : Sum  Inputs=+++++
  Clock1 : Clock
  Constant1 : Constant  Value="[0  -2/3*pi   2/3*pi]"
  Constant2 : Constant  Value=0
  Constant3 : Constant  Value=0
  Constant4 : Constant  Value=Pmax(3)
  Constant5 : Constant  Value=Pmin(3)
  Constant6 : Constant  Value=deg(3)
  Gain : Gain  Gain=kp(3)
  Gain1 : Gain  Gain=[1 1 1]
  Gain2 : Gain  Gain=120*pi*[1 1 1]
  Gain3 : Gain  Gain=V_m(3)
  Gain4 : Gain  Gain=1/P_base(3)
  Gain5 : Gain  Gain=[1 1 1]
  Gain6 : Gain  Gain=-1
  Gain7 : Gain  Gain=[1 1 1]
  Integrator : Integrator
  Product : Product
  Product1 : Product
  Scope1 : Scope
  Scope2 : Scope
  Scope3 : Scope
  Step : Step  Time=5  SampleTime=0
  Step1 : Step  Time=5  SampleTime=0
  Sum : Sum  Inputs=|+-
  Sum1 : Sum  Inputs=|+-
  Sum2 : Sum  Inputs=|++
  Switch : Switch  Criteria=u2 > Threshold  Threshold=Pmax(3)  SaturateOnIntegerOverflow=off  InputSameDT=off
  Switch1 : Switch  Criteria=u2 > Threshold  Threshold=-Pmin(3)  SaturateOnIntegerOverflow=off  InputSameDT=off
  Trigonometric Function1 : Trigonometry
  Out1 : Outport
  Out2 : Outport  Port=2
  wires:
  Clock1/1 -> Gain2/1
  Constant1/1 -> Add1/2
  Gain2/1 -> Add1/1
  Add1/1 -> Trigonometric Function1/1
  Gain1/1 -> Product/1
  Step/1 -> Product/2
  Product/1 -> Add1/3
  Trigonometric Function1/1 -> Gain3/1
  Gain3/1 -> Out1/1
  Gain/1 -> Scope2/1, Gain1/1
  Integrator/1 -> Gain/1
  P2/1 -> Gain4/1
  delta/1 -> Gain5/1
  Gain5/1 -> Add1/4
  Step1/1 -> Product1/2
  Product1/1 -> Integrator/1
  Constant4/1 -> Sum/1
  Sum/1 -> Switch/1
  Constant2/1 -> Switch/3
  Constant5/1 -> Sum1/1
  Sum1/1 -> Switch1/1
  Gain4/1 -> Gain6/1, Sum1/2, Sum/2, Switch/2
  Constant3/1 -> Switch1/3
  Gain6/1 -> Switch1/2
  Switch/1 -> Scope1/1, Sum2/1
  Switch1/1 -> Scope3/1, Sum2/2
  Sum2/1 -> Out2/1, Product1/1
  Constant6/1 -> Gain7/1
  Gain7/1 -> Add1/5

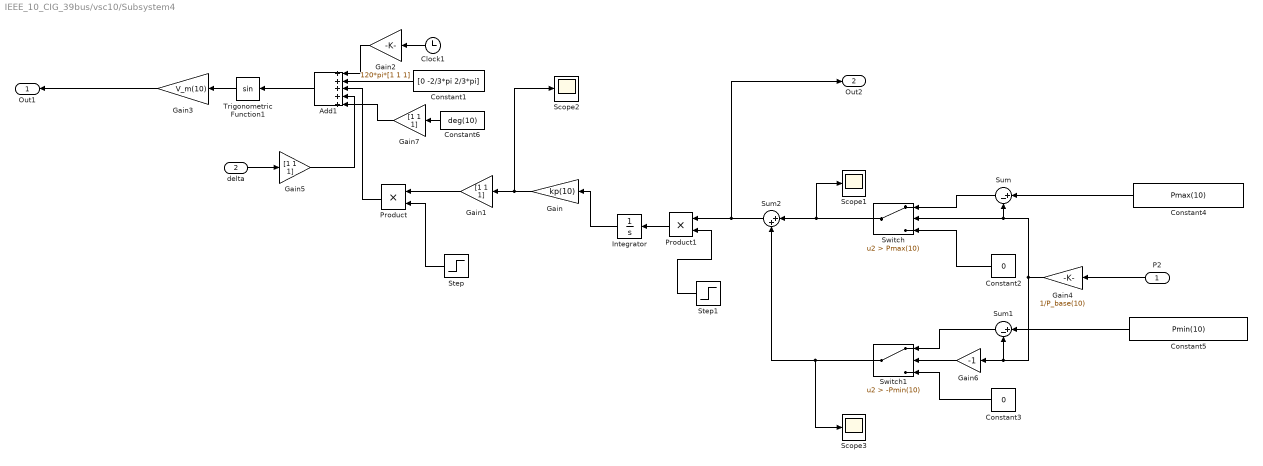
== system IEEE_10_CIG_39bus/vsc10/Subsystem4 ==
  P2 : Inport
  delta : Inport  Port=2
  Add1 : Sum  Inputs=+++++
  Clock1 : Clock
  Constant1 : Constant  Value="[0  -2/3*pi   2/3*pi]"
  Constant2 : Constant  Value=0
  Constant3 : Constant  Value=0
  Constant4 : Constant  Value=Pmax(10)
  Constant5 : Constant  Value=Pmin(10)
  Constant6 : Constant  Value=deg(10)
  Gain : Gain  Gain=kp(10)
  Gain1 : Gain  Gain=[1 1 1]
  Gain2 : Gain  Gain=120*pi*[1 1 1]
  Gain3 : Gain  Gain=V_m(10)
  Gain4 : Gain  Gain=1/P_base(10)
  Gain5 : Gain  Gain=[1 1 1]
  Gain6 : Gain  Gain=-1
  Gain7 : Gain  Gain=[1 1 1]
  Integrator : Integrator
  Product : Product
  Product1 : Product
  Scope1 : Scope
  Scope2 : Scope
  Scope3 : Scope
  Step : Step  Time=5  SampleTime=0
  Step1 : Step  Time=5  SampleTime=0
  Sum : Sum  Inputs=|+-
  Sum1 : Sum  Inputs=|+-
  Sum2 : Sum  Inputs=|++
  Switch : Switch  Criteria=u2 > Threshold  Threshold=Pmax(10)  SaturateOnIntegerOverflow=off  InputSameDT=off
  Switch1 : Switch  Criteria=u2 > Threshold  Threshold=-Pmin(10)  SaturateOnIntegerOverflow=off  InputSameDT=off
  Trigonometric Function1 : Trigonometry
  Out1 : Outport
  Out2 : Outport  Port=2
  wires:
  Clock1/1 -> Gain2/1
  Constant1/1 -> Add1/2
  Gain2/1 -> Add1/1
  Add1/1 -> Trigonometric Function1/1
  Gain1/1 -> Product/1
  Step/1 -> Product/2
  Product/1 -> Add1/3
  Trigonometric Function1/1 -> Gain3/1
  Gain3/1 -> Out1/1
  Gain/1 -> Scope2/1, Gain1/1
  Integrator/1 -> Gain/1
  P2/1 -> Gain4/1
  delta/1 -> Gain5/1
  Gain5/1 -> Add1/4
  Step1/1 -> Product1/2
  Product1/1 -> Integrator/1
  Constant4/1 -> Sum/1
  Sum/1 -> Switch/1
  Constant2/1 -> Switch/3
  Constant5/1 -> Sum1/1
  Sum1/1 -> Switch1/1
  Gain4/1 -> Gain6/1, Sum1/2, Sum/2, Switch/2
  Constant3/1 -> Switch1/3
  Gain6/1 -> Switch1/2
  Switch/1 -> Scope1/1, Sum2/1
  Switch1/1 -> Scope3/1, Sum2/2
  Sum2/1 -> Out2/1, Product1/1
  Constant6/1 -> Gain7/1
  Gain7/1 -> Add1/5

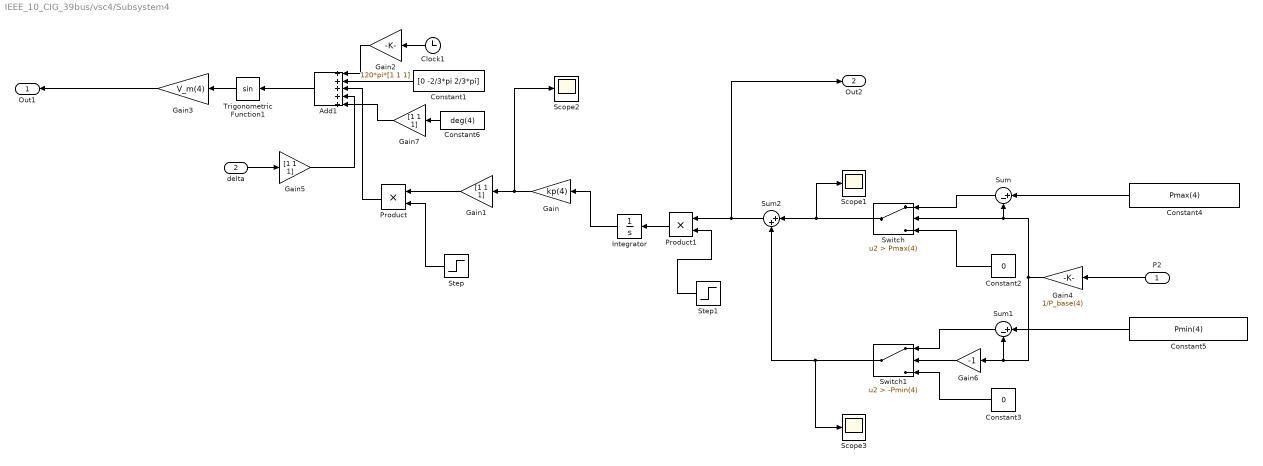
== system IEEE_10_CIG_39bus/vsc4/Subsystem4 ==
  P2 : Inport
  delta : Inport  Port=2
  Add1 : Sum  Inputs=+++++
  Clock1 : Clock
  Constant1 : Constant  Value="[0  -2/3*pi   2/3*pi]"
  Constant2 : Constant  Value=0
  Constant3 : Constant  Value=0
  Constant4 : Constant  Value=Pmax(4)
  Constant5 : Constant  Value=Pmin(4)
  Constant6 : Constant  Value=deg(4)
  Gain : Gain  Gain=kp(4)
  Gain1 : Gain  Gain=[1 1 1]
  Gain2 : Gain  Gain=120*pi*[1 1 1]
  Gain3 : Gain  Gain=V_m(4)
  Gain4 : Gain  Gain=1/P_base(4)
  Gain5 : Gain  Gain=[1 1 1]
  Gain6 : Gain  Gain=-1
  Gain7 : Gain  Gain=[1 1 1]
  Integrator : Integrator
  Product : Product
  Product1 : Product
  Scope1 : Scope
  Scope2 : Scope
  Scope3 : Scope
  Step : Step  Time=5  SampleTime=0
  Step1 : Step  Time=5  SampleTime=0
  Sum : Sum  Inputs=|+-
  Sum1 : Sum  Inputs=|+-
  Sum2 : Sum  Inputs=|++
  Switch : Switch  Criteria=u2 > Threshold  Threshold=Pmax(4)  SaturateOnIntegerOverflow=off  InputSameDT=off
  Switch1 : Switch  Criteria=u2 > Threshold  Threshold=-Pmin(4)  SaturateOnIntegerOverflow=off  InputSameDT=off
  Trigonometric Function1 : Trigonometry
  Out1 : Outport
  Out2 : Outport  Port=2
  wires:
  Clock1/1 -> Gain2/1
  Constant1/1 -> Add1/2
  Gain2/1 -> Add1/1
  Add1/1 -> Trigonometric Function1/1
  Gain1/1 -> Product/1
  Step/1 -> Product/2
  Product/1 -> Add1/3
  Trigonometric Function1/1 -> Gain3/1
  Gain3/1 -> Out1/1
  Gain/1 -> Scope2/1, Gain1/1
  Integrator/1 -> Gain/1
  P2/1 -> Gain4/1
  delta/1 -> Gain5/1
  Gain5/1 -> Add1/4
  Step1/1 -> Product1/2
  Product1/1 -> Integrator/1
  Constant4/1 -> Sum/1
  Sum/1 -> Switch/1
  Constant2/1 -> Switch/3
  Constant5/1 -> Sum1/1
  Sum1/1 -> Switch1/1
  Gain4/1 -> Gain6/1, Sum1/2, Sum/2, Switch/2
  Constant3/1 -> Switch1/3
  Gain6/1 -> Switch1/2
  Switch/1 -> Scope1/1, Sum2/1
  Switch1/1 -> Scope3/1, Sum2/2
  Sum2/1 -> Out2/1, Product1/1
  Constant6/1 -> Gain7/1
  Gain7/1 -> Add1/5

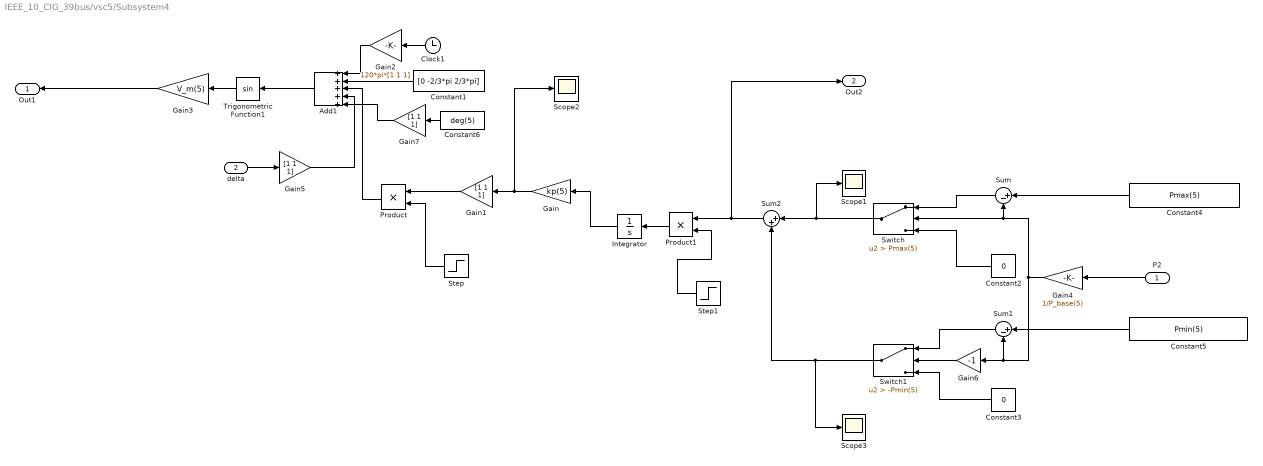
== system IEEE_10_CIG_39bus/vsc5/Subsystem4 ==
  P2 : Inport
  delta : Inport  Port=2
  Add1 : Sum  Inputs=+++++
  Clock1 : Clock
  Constant1 : Constant  Value="[0  -2/3*pi   2/3*pi]"
  Constant2 : Constant  Value=0
  Constant3 : Constant  Value=0
  Constant4 : Constant  Value=Pmax(5)
  Constant5 : Constant  Value=Pmin(5)
  Constant6 : Constant  Value=deg(5)
  Gain : Gain  Gain=kp(5)
  Gain1 : Gain  Gain=[1 1 1]
  Gain2 : Gain  Gain=120*pi*[1 1 1]
  Gain3 : Gain  Gain=V_m(5)
  Gain4 : Gain  Gain=1/P_base(5)
  Gain5 : Gain  Gain=[1 1 1]
  Gain6 : Gain  Gain=-1
  Gain7 : Gain  Gain=[1 1 1]
  Integrator : Integrator
  Product : Product
  Product1 : Product
  Scope1 : Scope
  Scope2 : Scope
  Scope3 : Scope
  Step : Step  Time=5  SampleTime=0
  Step1 : Step  Time=5  SampleTime=0
  Sum : Sum  Inputs=|+-
  Sum1 : Sum  Inputs=|+-
  Sum2 : Sum  Inputs=|++
  Switch : Switch  Criteria=u2 > Threshold  Threshold=Pmax(5)  SaturateOnIntegerOverflow=off  InputSameDT=off
  Switch1 : Switch  Criteria=u2 > Threshold  Threshold=-Pmin(5)  SaturateOnIntegerOverflow=off  InputSameDT=off
  Trigonometric Function1 : Trigonometry
  Out1 : Outport
  Out2 : Outport  Port=2
  wires:
  Clock1/1 -> Gain2/1
  Constant1/1 -> Add1/2
  Gain2/1 -> Add1/1
  Add1/1 -> Trigonometric Function1/1
  Gain1/1 -> Product/1
  Step/1 -> Product/2
  Product/1 -> Add1/3
  Trigonometric Function1/1 -> Gain3/1
  Gain3/1 -> Out1/1
  Gain/1 -> Scope2/1, Gain1/1
  Integrator/1 -> Gain/1
  P2/1 -> Gain4/1
  delta/1 -> Gain5/1
  Gain5/1 -> Add1/4
  Step1/1 -> Product1/2
  Product1/1 -> Integrator/1
  Constant4/1 -> Sum/1
  Sum/1 -> Switch/1
  Constant2/1 -> Switch/3
  Constant5/1 -> Sum1/1
  Sum1/1 -> Switch1/1
  Gain4/1 -> Gain6/1, Sum1/2, Sum/2, Switch/2
  Constant3/1 -> Switch1/3
  Gain6/1 -> Switch1/2
  Switch/1 -> Scope1/1, Sum2/1
  Switch1/1 -> Scope3/1, Sum2/2
  Sum2/1 -> Out2/1, Product1/1
  Constant6/1 -> Gain7/1
  Gain7/1 -> Add1/5

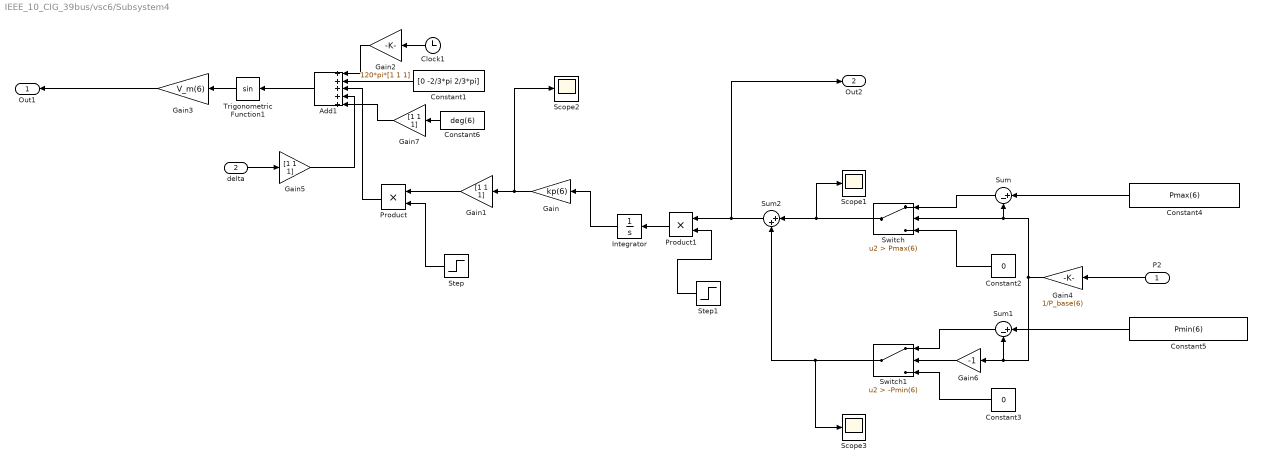
== system IEEE_10_CIG_39bus/vsc6/Subsystem4 ==
  P2 : Inport
  delta : Inport  Port=2
  Add1 : Sum  Inputs=+++++
  Clock1 : Clock
  Constant1 : Constant  Value="[0  -2/3*pi   2/3*pi]"
  Constant2 : Constant  Value=0
  Constant3 : Constant  Value=0
  Constant4 : Constant  Value=Pmax(6)
  Constant5 : Constant  Value=Pmin(6)
  Constant6 : Constant  Value=deg(6)
  Gain : Gain  Gain=kp(6)
  Gain1 : Gain  Gain=[1 1 1]
  Gain2 : Gain  Gain=120*pi*[1 1 1]
  Gain3 : Gain  Gain=V_m(6)
  Gain4 : Gain  Gain=1/P_base(6)
  Gain5 : Gain  Gain=[1 1 1]
  Gain6 : Gain  Gain=-1
  Gain7 : Gain  Gain=[1 1 1]
  Integrator : Integrator
  Product : Product
  Product1 : Product
  Scope1 : Scope
  Scope2 : Scope
  Scope3 : Scope
  Step : Step  Time=5  SampleTime=0
  Step1 : Step  Time=5  SampleTime=0
  Sum : Sum  Inputs=|+-
  Sum1 : Sum  Inputs=|+-
  Sum2 : Sum  Inputs=|++
  Switch : Switch  Criteria=u2 > Threshold  Threshold=Pmax(6)  SaturateOnIntegerOverflow=off  InputSameDT=off
  Switch1 : Switch  Criteria=u2 > Threshold  Threshold=-Pmin(6)  SaturateOnIntegerOverflow=off  InputSameDT=off
  Trigonometric Function1 : Trigonometry
  Out1 : Outport
  Out2 : Outport  Port=2
  wires:
  Clock1/1 -> Gain2/1
  Constant1/1 -> Add1/2
  Gain2/1 -> Add1/1
  Add1/1 -> Trigonometric Function1/1
  Gain1/1 -> Product/1
  Step/1 -> Product/2
  Product/1 -> Add1/3
  Trigonometric Function1/1 -> Gain3/1
  Gain3/1 -> Out1/1
  Gain/1 -> Scope2/1, Gain1/1
  Integrator/1 -> Gain/1
  P2/1 -> Gain4/1
  delta/1 -> Gain5/1
  Gain5/1 -> Add1/4
  Step1/1 -> Product1/2
  Product1/1 -> Integrator/1
  Constant4/1 -> Sum/1
  Sum/1 -> Switch/1
  Constant2/1 -> Switch/3
  Constant5/1 -> Sum1/1
  Sum1/1 -> Switch1/1
  Gain4/1 -> Gain6/1, Sum1/2, Sum/2, Switch/2
  Constant3/1 -> Switch1/3
  Gain6/1 -> Switch1/2
  Switch/1 -> Scope1/1, Sum2/1
  Switch1/1 -> Scope3/1, Sum2/2
  Sum2/1 -> Out2/1, Product1/1
  Constant6/1 -> Gain7/1
  Gain7/1 -> Add1/5

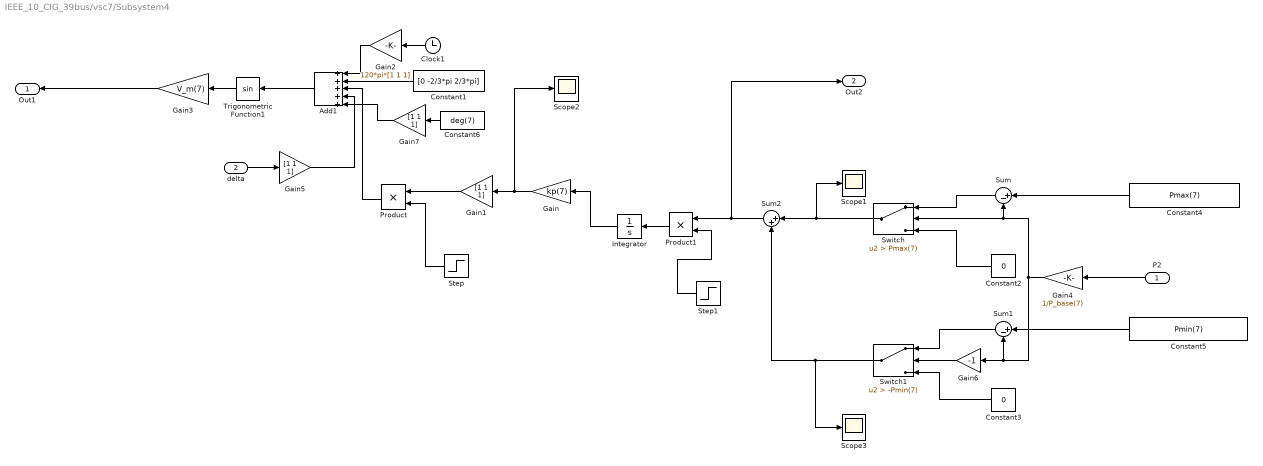
== system IEEE_10_CIG_39bus/vsc7/Subsystem4 ==
  P2 : Inport
  delta : Inport  Port=2
  Add1 : Sum  Inputs=+++++
  Clock1 : Clock
  Constant1 : Constant  Value="[0  -2/3*pi   2/3*pi]"
  Constant2 : Constant  Value=0
  Constant3 : Constant  Value=0
  Constant4 : Constant  Value=Pmax(7)
  Constant5 : Constant  Value=Pmin(7)
  Constant6 : Constant  Value=deg(7)
  Gain : Gain  Gain=kp(7)
  Gain1 : Gain  Gain=[1 1 1]
  Gain2 : Gain  Gain=120*pi*[1 1 1]
  Gain3 : Gain  Gain=V_m(7)
  Gain4 : Gain  Gain=1/P_base(7)
  Gain5 : Gain  Gain=[1 1 1]
  Gain6 : Gain  Gain=-1
  Gain7 : Gain  Gain=[1 1 1]
  Integrator : Integrator
  Product : Product
  Product1 : Product
  Scope1 : Scope
  Scope2 : Scope
  Scope3 : Scope
  Step : Step  Time=5  SampleTime=0
  Step1 : Step  Time=5  SampleTime=0
  Sum : Sum  Inputs=|+-
  Sum1 : Sum  Inputs=|+-
  Sum2 : Sum  Inputs=|++
  Switch : Switch  Criteria=u2 > Threshold  Threshold=Pmax(7)  SaturateOnIntegerOverflow=off  InputSameDT=off
  Switch1 : Switch  Criteria=u2 > Threshold  Threshold=-Pmin(7)  SaturateOnIntegerOverflow=off  InputSameDT=off
  Trigonometric Function1 : Trigonometry
  Out1 : Outport
  Out2 : Outport  Port=2
  wires:
  Clock1/1 -> Gain2/1
  Constant1/1 -> Add1/2
  Gain2/1 -> Add1/1
  Add1/1 -> Trigonometric Function1/1
  Gain1/1 -> Product/1
  Step/1 -> Product/2
  Product/1 -> Add1/3
  Trigonometric Function1/1 -> Gain3/1
  Gain3/1 -> Out1/1
  Gain/1 -> Scope2/1, Gain1/1
  Integrator/1 -> Gain/1
  P2/1 -> Gain4/1
  delta/1 -> Gain5/1
  Gain5/1 -> Add1/4
  Step1/1 -> Product1/2
  Product1/1 -> Integrator/1
  Constant4/1 -> Sum/1
  Sum/1 -> Switch/1
  Constant2/1 -> Switch/3
  Constant5/1 -> Sum1/1
  Sum1/1 -> Switch1/1
  Gain4/1 -> Gain6/1, Sum1/2, Sum/2, Switch/2
  Constant3/1 -> Switch1/3
  Gain6/1 -> Switch1/2
  Switch/1 -> Scope1/1, Sum2/1
  Switch1/1 -> Scope3/1, Sum2/2
  Sum2/1 -> Out2/1, Product1/1
  Constant6/1 -> Gain7/1
  Gain7/1 -> Add1/5

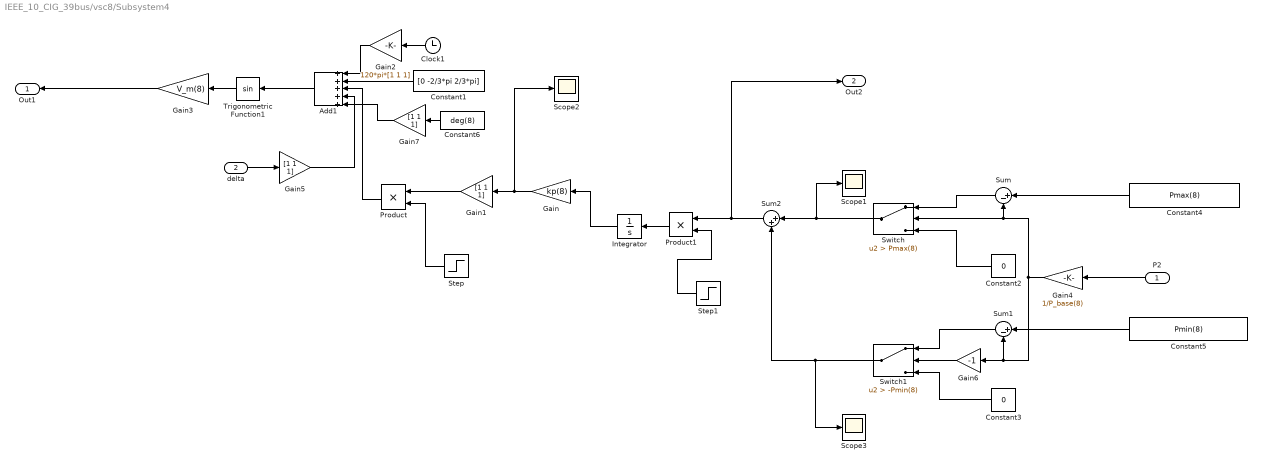
== system IEEE_10_CIG_39bus/vsc8/Subsystem4 ==
  P2 : Inport
  delta : Inport  Port=2
  Add1 : Sum  Inputs=+++++
  Clock1 : Clock
  Constant1 : Constant  Value="[0  -2/3*pi   2/3*pi]"
  Constant2 : Constant  Value=0
  Constant3 : Constant  Value=0
  Constant4 : Constant  Value=Pmax(8)
  Constant5 : Constant  Value=Pmin(8)
  Constant6 : Constant  Value=deg(8)
  Gain : Gain  Gain=kp(8)
  Gain1 : Gain  Gain=[1 1 1]
  Gain2 : Gain  Gain=120*pi*[1 1 1]
  Gain3 : Gain  Gain=V_m(8)
  Gain4 : Gain  Gain=1/P_base(8)
  Gain5 : Gain  Gain=[1 1 1]
  Gain6 : Gain  Gain=-1
  Gain7 : Gain  Gain=[1 1 1]
  Integrator : Integrator
  Product : Product
  Product1 : Product
  Scope1 : Scope
  Scope2 : Scope
  Scope3 : Scope
  Step : Step  Time=5  SampleTime=0
  Step1 : Step  Time=5  SampleTime=0
  Sum : Sum  Inputs=|+-
  Sum1 : Sum  Inputs=|+-
  Sum2 : Sum  Inputs=|++
  Switch : Switch  Criteria=u2 > Threshold  Threshold=Pmax(8)  SaturateOnIntegerOverflow=off  InputSameDT=off
  Switch1 : Switch  Criteria=u2 > Threshold  Threshold=-Pmin(8)  SaturateOnIntegerOverflow=off  InputSameDT=off
  Trigonometric Function1 : Trigonometry
  Out1 : Outport
  Out2 : Outport  Port=2
  wires:
  Clock1/1 -> Gain2/1
  Constant1/1 -> Add1/2
  Gain2/1 -> Add1/1
  Add1/1 -> Trigonometric Function1/1
  Gain1/1 -> Product/1
  Step/1 -> Product/2
  Product/1 -> Add1/3
  Trigonometric Function1/1 -> Gain3/1
  Gain3/1 -> Out1/1
  Gain/1 -> Scope2/1, Gain1/1
  Integrator/1 -> Gain/1
  P2/1 -> Gain4/1
  delta/1 -> Gain5/1
  Gain5/1 -> Add1/4
  Step1/1 -> Product1/2
  Product1/1 -> Integrator/1
  Constant4/1 -> Sum/1
  Sum/1 -> Switch/1
  Constant2/1 -> Switch/3
  Constant5/1 -> Sum1/1
  Sum1/1 -> Switch1/1
  Gain4/1 -> Gain6/1, Sum1/2, Sum/2, Switch/2
  Constant3/1 -> Switch1/3
  Gain6/1 -> Switch1/2
  Switch/1 -> Scope1/1, Sum2/1
  Switch1/1 -> Scope3/1, Sum2/2
  Sum2/1 -> Out2/1, Product1/1
  Constant6/1 -> Gain7/1
  Gain7/1 -> Add1/5

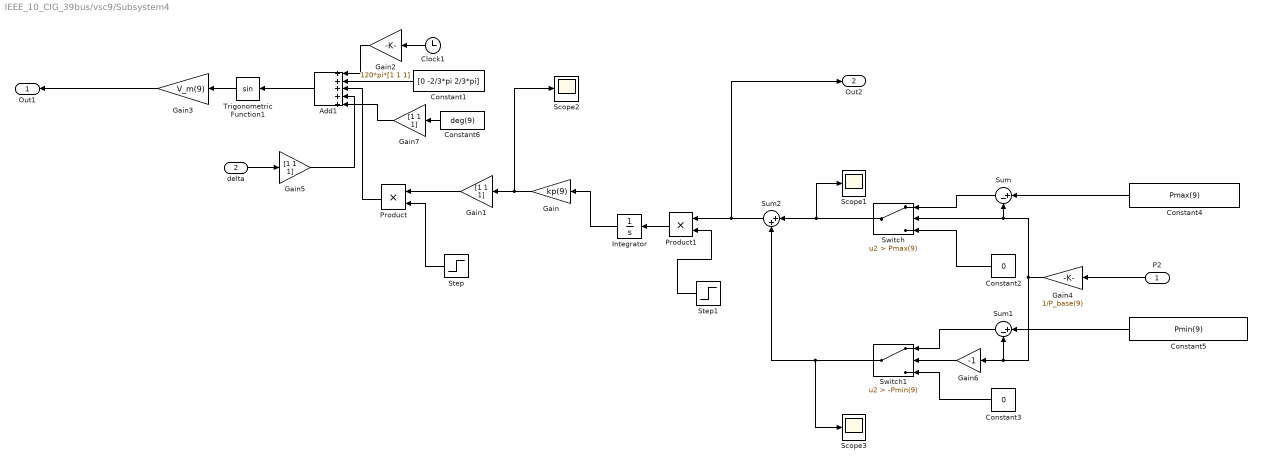
== system IEEE_10_CIG_39bus/vsc9/Subsystem4 ==
  P2 : Inport
  delta : Inport  Port=2
  Add1 : Sum  Inputs=+++++
  Clock1 : Clock
  Constant1 : Constant  Value="[0  -2/3*pi   2/3*pi]"
  Constant2 : Constant  Value=0
  Constant3 : Constant  Value=0
  Constant4 : Constant  Value=Pmax(9)
  Constant5 : Constant  Value=Pmin(9)
  Constant6 : Constant  Value=deg(9)
  Gain : Gain  Gain=kp(9)
  Gain1 : Gain  Gain=[1 1 1]
  Gain2 : Gain  Gain=120*pi*[1 1 1]
  Gain3 : Gain  Gain=V_m(9)
  Gain4 : Gain  Gain=1/P_base(9)
  Gain5 : Gain  Gain=[1 1 1]
  Gain6 : Gain  Gain=-1
  Gain7 : Gain  Gain=[1 1 1]
  Integrator : Integrator
  Product : Product
  Product1 : Product
  Scope1 : Scope
  Scope2 : Scope
  Scope3 : Scope
  Step : Step  Time=5  SampleTime=0
  Step1 : Step  Time=5  SampleTime=0
  Sum : Sum  Inputs=|+-
  Sum1 : Sum  Inputs=|+-
  Sum2 : Sum  Inputs=|++
  Switch : Switch  Criteria=u2 > Threshold  Threshold=Pmax(9)  SaturateOnIntegerOverflow=off  InputSameDT=off
  Switch1 : Switch  Criteria=u2 > Threshold  Threshold=-Pmin(9)  SaturateOnIntegerOverflow=off  InputSameDT=off
  Trigonometric Function1 : Trigonometry
  Out1 : Outport
  Out2 : Outport  Port=2
  wires:
  Clock1/1 -> Gain2/1
  Constant1/1 -> Add1/2
  Gain2/1 -> Add1/1
  Add1/1 -> Trigonometric Function1/1
  Gain1/1 -> Product/1
  Step/1 -> Product/2
  Product/1 -> Add1/3
  Trigonometric Function1/1 -> Gain3/1
  Gain3/1 -> Out1/1
  Gain/1 -> Scope2/1, Gain1/1
  Integrator/1 -> Gain/1
  P2/1 -> Gain4/1
  delta/1 -> Gain5/1
  Gain5/1 -> Add1/4
  Step1/1 -> Product1/2
  Product1/1 -> Integrator/1
  Constant4/1 -> Sum/1
  Sum/1 -> Switch/1
  Constant2/1 -> Switch/3
  Constant5/1 -> Sum1/1
  Sum1/1 -> Switch1/1
  Gain4/1 -> Gain6/1, Sum1/2, Sum/2, Switch/2
  Constant3/1 -> Switch1/3
  Gain6/1 -> Switch1/2
  Switch/1 -> Scope1/1, Sum2/1
  Switch1/1 -> Scope3/1, Sum2/2
  Sum2/1 -> Out2/1, Product1/1
  Constant6/1 -> Gain7/1
  Gain7/1 -> Add1/5
